simulink model "aircraft_control_model_v2"  (R2020b)
settings: Solver=ode1be  StartTime=0.0  StopTime=t  RelTol=1e-3
values from neighbouring files (symbols this model uses):
  A_ce_CG_14 = A_ce_CG_14(2:3,2:3)    [aircraft_control_model_initialisation_v2.m]
  A_ce_CG_24 = A_ce_CG_24(2:3,2:3)    [aircraft_control_model_initialisation_v2.m]
  A_ce_CG_34 = A_ce_CG_34(2:3,2:3)    [aircraft_control_model_initialisation_v2.m]
  A_sc_CG_10 = A_sc_CG_10(2:3,2:3)    [aircraft_control_model_initialisation_v2.m]
  A_sc_CG_22 = A_sc_CG_22(2:3,2:3)    [aircraft_control_model_initialisation_v2.m]
  A_sc_CG_29 = A_sc_CG_29(2:3,2:3)    [aircraft_control_model_initialisation_v2.m]
  A_sc_CG_36 = A_sc_CG_36(2:3,2:3)    [aircraft_control_model_initialisation_v2.m]
  A_sc_CG_55 = A_sc_CG_55(2:3,2:3)    [aircraft_control_model_initialisation_v2.m]
  actuator_rate = 115*pi/180    (= 2.00712863979)    [aircraft_control_model_initialisation_v2.m]
  ail_sat = 30*pi/180    (= 0.523598775598)    [aircraft_control_model_initialisation_v2.m]
  alpha0 = base_scout_aircraft_constants(16)    [aircraft_control_model_initialisation_v2.m]
  alpha0_ce = base_cessna_aircraft_constants(16)    [aircraft_control_model_initialisation_v2.m]
  alpha0tot_ce_CG_14 = consts_ce_CG_14(17)    [aircraft_control_model_initialisation_v2.m]
  alpha0tot_ce_CG_24 = consts_ce_CG_24(17)    [aircraft_control_model_initialisation_v2.m]
  alpha0tot_ce_CG_34 = consts_ce_CG_34(17)    [aircraft_control_model_initialisation_v2.m]
  alpha0tot_sc_CG_10 = consts_sc_CG_10(17)    [aircraft_control_model_initialisation_v2.m]
  alpha0tot_sc_CG_22 = consts_sc_CG_22(17)    [aircraft_control_model_initialisation_v2.m]
  alpha0tot_sc_CG_29 = consts_sc_CG_29(17)    [aircraft_control_model_initialisation_v2.m]
  alpha0tot_sc_CG_36 = consts_sc_CG_36(17)    [aircraft_control_model_initialisation_v2.m]
  alpha0tot_sc_CG_55 = consts_sc_CG_55(17)    [aircraft_control_model_initialisation_v2.m]
  alpha_ts = base_scout_aircraft_constants(19)    [aircraft_control_model_initialisation_v2.m]
  alpha_ts_ce = base_cessna_aircraft_constants(19)    [aircraft_control_model_initialisation_v2.m]
  alpha_ws = base_scout_aircraft_constants(18)    [aircraft_control_model_initialisation_v2.m]
  alpha_ws_ce = base_cessna_aircraft_constants(18)    [aircraft_control_model_initialisation_v2.m]
  AR_w = base_scout_aircraft_constants(8)    [aircraft_control_model_initialisation_v2.m]
  AR_w_ce = base_cessna_aircraft_constants(8)    [aircraft_control_model_initialisation_v2.m]
  b1 = base_scout_aircraft_constants(23)    [aircraft_control_model_initialisation_v2.m]
  b1_ce = base_cessna_aircraft_constants(23)    [aircraft_control_model_initialisation_v2.m]
  b2 = base_scout_aircraft_constants(24)    [aircraft_control_model_initialisation_v2.m]
  b2_ce = base_cessna_aircraft_constants(24)    [aircraft_control_model_initialisation_v2.m]
  b3 = base_scout_aircraft_constants(25)    [aircraft_control_model_initialisation_v2.m]
  b3_ce = base_cessna_aircraft_constants(25)    [aircraft_control_model_initialisation_v2.m]
  B_ce_CG_14 = B_ce_CG_14(2:3,1:1)    [aircraft_control_model_initialisation_v2.m]
  B_ce_CG_24 = B_ce_CG_24(2:3,1:1)    [aircraft_control_model_initialisation_v2.m]
  B_ce_CG_34 = B_ce_CG_34(2:3,1:1)    [aircraft_control_model_initialisation_v2.m]
  B_sc = B_sc(:,1)    [aircraft_control_model_initialisation_v2.m]
  B_sc_CG_10 = B_sc_CG_10(2:3,1:1)    [aircraft_control_model_initialisation_v2.m]
  B_sc_CG_22 = B_sc_CG_22(2:3,1:1)    [aircraft_control_model_initialisation_v2.m]
  B_sc_CG_29 = B_sc_CG_29(2:3,1:1)    [aircraft_control_model_initialisation_v2.m]
  B_sc_CG_36 = B_sc_CG_36(2:3,1:1)    [aircraft_control_model_initialisation_v2.m]
  B_sc_CG_55 = B_sc_CG_55(2:3,1:1)    [aircraft_control_model_initialisation_v2.m]
  beta_ce_CG_14 = consts_ce_CG_14(21)    [aircraft_control_model_initialisation_v2.m]
  beta_ce_CG_24 = consts_ce_CG_24(21)    [aircraft_control_model_initialisation_v2.m]
  beta_ce_CG_34 = consts_ce_CG_34(21)    [aircraft_control_model_initialisation_v2.m]
  beta_sc_CG_10 = consts_sc_CG_10(21)    [aircraft_control_model_initialisation_v2.m]
  beta_sc_CG_22 = consts_sc_CG_22(21)    [aircraft_control_model_initialisation_v2.m]
  beta_sc_CG_29 = consts_sc_CG_29(21)    [aircraft_control_model_initialisation_v2.m]
  beta_sc_CG_36 = consts_sc_CG_36(21)    [aircraft_control_model_initialisation_v2.m]
  beta_sc_CG_55 = consts_sc_CG_55(21)    [aircraft_control_model_initialisation_v2.m]
  c_e = base_scout_aircraft_constants(10)    [aircraft_control_model_initialisation_v2.m]
  c_e_ce = base_cessna_aircraft_constants(10)    [aircraft_control_model_initialisation_v2.m]
  Cm0 = base_scout_aircraft_constants(11)    [aircraft_control_model_initialisation_v2.m]
  control_surface_feedback = 10    [aircraft_control_model_initialisation_v2.m]
  dCL_w_dalpha = base_scout_aircraft_constants(14)    [aircraft_control_model_initialisation_v2.m]
  dCL_w_dalpha_ce = base_cessna_aircraft_constants(14)    [aircraft_control_model_initialisation_v2.m]
  dCLtot_dalpha = base_scout_aircraft_constants(15)    [aircraft_control_model_initialisation_v2.m]
  dCLtot_dalpha_ce = base_cessna_aircraft_constants(15)    [aircraft_control_model_initialisation_v2.m]
  dt = 1/100    (= 0.01)    [aircraft_control_model_initialisation_v2.m]
  elev_amplitude = 15*pi/180    (= 0.261799387799)    [aircraft_control_model_initialisation_v2.m]
  elev_cutoff = 35*pi/180    (= 0.610865238198)    [aircraft_control_model_initialisation_v2.m]
  elev_period = 1    [aircraft_control_model_initialisation_v2.m]
  elev_period_start = 5    [aircraft_control_model_initialisation_v2.m]
  elev_sat = 28*pi/180    (= 0.488692190558)    [aircraft_control_model_initialisation_v2.m]
  eta_ce_CG_14 = consts_ce_CG_14(22)    [aircraft_control_model_initialisation_v2.m]
  eta_ce_CG_24 = consts_ce_CG_24(22)    [aircraft_control_model_initialisation_v2.m]
  eta_ce_CG_34 = consts_ce_CG_34(22)    [aircraft_control_model_initialisation_v2.m]
  eta_sc_CG_10 = consts_sc_CG_10(22)    [aircraft_control_model_initialisation_v2.m]
  eta_sc_CG_22 = consts_sc_CG_22(22)    [aircraft_control_model_initialisation_v2.m]
  eta_sc_CG_29 = consts_sc_CG_29(22)    [aircraft_control_model_initialisation_v2.m]
  eta_sc_CG_36 = consts_sc_CG_36(22)    [aircraft_control_model_initialisation_v2.m]
  eta_sc_CG_55 = consts_sc_CG_55(22)    [aircraft_control_model_initialisation_v2.m]
  g = base_scout_aircraft_constants(3)    [aircraft_control_model_initialisation_v2.m]
  G = base_scout_aircraft_constants(26)    [aircraft_control_model_initialisation_v2.m]
  g_ce = base_cessna_aircraft_constants(3)    [aircraft_control_model_initialisation_v2.m]
  G_ce = base_cessna_aircraft_constants(26)    [aircraft_control_model_initialisation_v2.m]
  h0 = base_scout_aircraft_constants(13)    [aircraft_control_model_initialisation_v2.m]
  h_cg = base_scout_aircraft_constants(12)    [aircraft_control_model_initialisation_v2.m]
  K = base_scout_aircraft_constants(7)    [aircraft_control_model_initialisation_v2.m]
  l_m = base_scout_aircraft_constants(27)    [aircraft_control_model_initialisation_v2.m]
  l_m_ce = base_cessna_aircraft_constants(27)    [aircraft_control_model_initialisation_v2.m]
  m = base_scout_aircraft_constants(2)    [aircraft_control_model_initialisation_v2.m]
  m_ce = base_cessna_aircraft_constants(2)    [aircraft_control_model_initialisation_v2.m]
  modM = base_scout_aircraft_constants(30)    [aircraft_control_model_initialisation_v2.m]
  modM_ce = base_cessna_aircraft_constants(30)    [aircraft_control_model_initialisation_v2.m]
  n = base_scout_aircraft_constants(1)    [aircraft_control_model_initialisation_v2.m]    (also in xplane_data_decoder.m = data_input(6,2))
  ppgain_actuator_D = 1.076123507883140e+02    (= 107.612350788)    [aircraft_control_model_initialisation_v2.m]
  ppgain_actuator_P = 20.729870007825970    (= 20.7298700078)    [aircraft_control_model_initialisation_v2.m]
  ppgain_D = 0.637114873357555    (= 0.637114873358)    [aircraft_control_model_initialisation_v2.m]
  ppgain_P = -86.717674561182620    (= -86.7176745612)    [aircraft_control_model_initialisation_v2.m]
  r = base_scout_aircraft_constants(29)    [aircraft_control_model_initialisation_v2.m]
  r_ce = base_cessna_aircraft_constants(29)    [aircraft_control_model_initialisation_v2.m]
  rho = base_scout_aircraft_constants(4)    [aircraft_control_model_initialisation_v2.m]
  rho_ce = base_cessna_aircraft_constants(4)    [aircraft_control_model_initialisation_v2.m]
  rud_sat = 28*pi/180    (= 0.488692190558)    [aircraft_control_model_initialisation_v2.m]
  s_e = base_scout_aircraft_constants(9)    [aircraft_control_model_initialisation_v2.m]
  s_e_ce = base_cessna_aircraft_constants(9)    [aircraft_control_model_initialisation_v2.m]
  s_tp = base_scout_aircraft_constants(6)    [aircraft_control_model_initialisation_v2.m]
  s_w = base_scout_aircraft_constants(5)    [aircraft_control_model_initialisation_v2.m]
  s_w_ce = base_cessna_aircraft_constants(5)    [aircraft_control_model_initialisation_v2.m]
  tr = base_scout_aircraft_constants(28)    [aircraft_control_model_initialisation_v2.m]
  tr_ce = base_cessna_aircraft_constants(28)    [aircraft_control_model_initialisation_v2.m]
undefined symbols (not defined in the file or in its folder): A_sc
libraries: simulink x6, pid_lib x4, etargetslib x2, dspnetwork x2, aerolibanimutils x1, sldrtlib x1, cstblocks x1
(part 1 of 3)
settings Model: Creator=declan  LastModifiedBy=declan

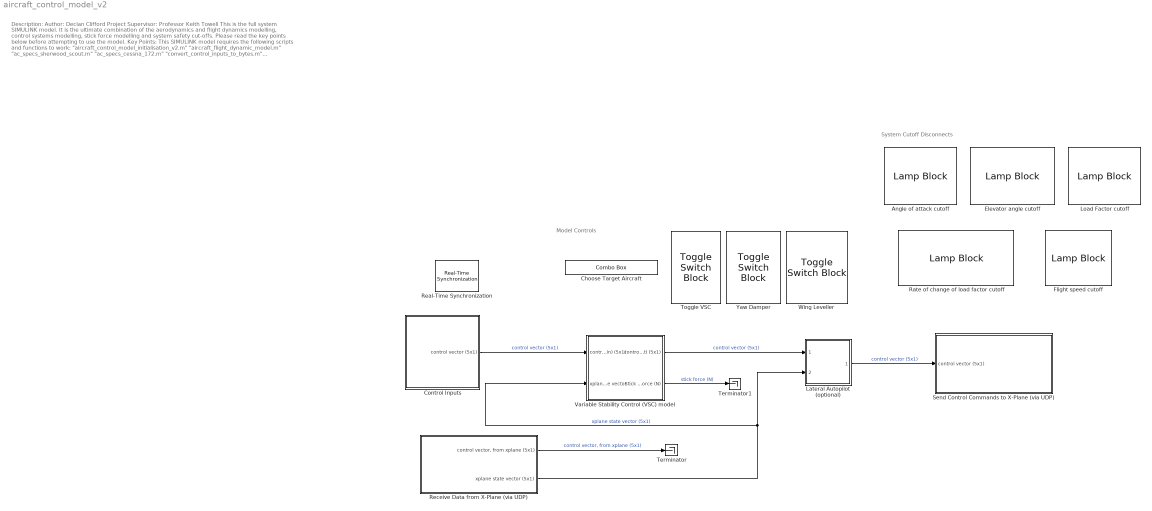
== system aircraft_control_model_v2 ==
  note: Description:
      |
      | Author: Declan Clifford
      | Project Supervisor: Professor Keith Towell
      |
      | This is the full system SIMULINK model. It is the ultimate combination of the aerodynamics and flight dynamics modelling, control systems modelling, stick force modelling and system safety cut-offs.
      |
      | Please read the key points below before attempting to use the model.
      |
      | Key Points:
      |
      | This SIMULINK model requires the following scripts and functions to work:
      | "aircraft_control_model_initialisation_v2.m"
      | "aircraft_flight_dynamic_model.m"
      | "ac_specs_sherwood_scout.m"
      | "ac_specs_cessna_172.m"
      | "convert_control_inputs_to_bytes.m"
      | "elevator_input.m"
      | "flightspeedcutoff.m"
      | "xplane_data_decoder.m"
      |
      | "aircraft_control_model_initialisation_v2" is the SIMULINK model's initialisation script. Please run this script before using the SIMULINK model. It is important the user reads and understand the initialisation script before using the SIMULINK model.
      |
      | "aircraft_flight_dynamic_model" generates the state space matrices required for the flight simulations in this SIMULINK model. It is important the user reads and understands this script before using the SIMULINK model.
      |
      | The model is integrated with X-Plane 11, version 11.52. Connection with X-Plane is performed via UDP. NOTE: USING DIFFERENT VERSIONS OF X-PLANE RUNS THE RISK OF THE RECEIVED DATA REFS BEING INCORRECT, AND SO NONE OF THE RECEIVED DATA FROM X-PLANE WILL BE CORRECT.
      |
      | The X-Plane 11 Sherwood Scout Model can be found at:
      | https://github.com/TheOfficialDarthVader/GDP_52_Variable_Stability_Demonstrator/tree/main/x_plane_sherwood_scout
      | There are three versions of this model; a version with struts, a version without struts and an older "legacy" version of the model.
      |
      | It is recommended to use the wing yaw damper and wing leveller while running X-Plane. This will allow the pilot to forget about lateral aircraft control and focus only on inputting elevator deflections. The throttle will still however need to be controlled to trim the aircraft.
      |
      | The model control inputs are either in the form of a USB joystick or predefined control input. See the "control inputs" block for more details. The joystick inputs for pitch, roll, yaw and the throttle should be quite universal, however the trim tab control has been set up as two button commands. button 6 and button 4.
      |
      | As it stands the model is fully functional, however some parts of it are unfinished. The model is currently tuned to work with only the rear actuator model. A front actuator model has not been integrated with this system. Due to unforeseen delays, the Volz servos front actuator model could not be linearsed and integrated with this system. The full, nonlinearised version of the Volz servos front actuator model slows the system down significantly as it is a separate SIMULINK model and so this was not a viable option.
      |
      | Two of the system safety cut-offs are likewise unfinished. These are the rate of change of load factor cutoff and the flight speed cutoff.
      | The rate of change of load factor cut-off can be implemented as follows:
      | At some time step, determine the rate of change of load factor required to cause the aircraft to exceed the load factor limit in some time interval, chosen as 0.1 seconds here. This is the rate of change of load factor cut-off.
      | In algebraic form this could be expressed as:
      | rate_of_change_of_load_factor_cutoff=(load_factor_limit-present_load_factor)/0.1
      | The rate of change of load factor cut-off currently implemented simply states the rate of change of load factor must not exceed 7.8g/s. The output of this cut-off has been multiplied by a gain of zero, which can be removed when the proper method has been implemeted
      |
      | The flight speed cut-off is half implemented. At present it will only cut-off the control system if the flight speed at a current load factor will cause the aircraft to stall. This is stall under both positive and negative g loading. This should very broadly be expanded to the entire flight envelope. So, if the aircraft's flight speed at the aircraft's current load factor is outside of the flight envelope, or very near it, the system should cut-off. As stated before, this has already been done for the stall limits. It's worth noting that the load factor cut-offs are fully functional and the control system will cut-off at a load factor of 3.8g and -0.5g. This is a separate cut-off to the flight speed cut-off.
  note: Model Controls
  note: System Cutoff Disconnects
  Angle of attack cutoff : LampBlock
  Choose Target Aircraft : ComboBox  LabelPosition=Hide  SelectedLabel=Scout CG 0.2935
      settings: Values={{'Scout CG 0.1', 'Scout CG 0.223', 'Scout CG 0.2935', 'Scout CG 0.364', 'Scout CG 0.55', 'Cessna Forward CG', 'Cessna Centre CG', 'Cessna Aft CG', '>:(', 'F-4C Phantom', 'B-747-100'}, [1 2 3 4 5 6 7 8 9 10 11]}
  Control Inputs : Subsystem  mask{controlvectorselect=Joystick}
      mask prompts: controlvectorselect "Select control method >:("
      mask TypeOptions controlvectorselect: Predefined Input | Joystick
      mask Display: image('control_inputs.JPG'); % Use "Edit Image" on toolstrip to change.
  Elevator angle cutoff : LampBlock
  Flight speed cutoff : LampBlock
  Lateral Autopilot (optional) : Subsystem
      mask Display: image('autopilot_symbol.JPG'); % Use "Edit Image" on toolstrip to change.
  Load Factor cutoff : LampBlock
  Rate of change of load factor cutoff : LampBlock
  Real-Time Synchronization : sldrtlib/Real-Time Synchronization  SampleTime=dt  MaxMissedTicks=500  ShowMissedTicks=off  YieldWhenWaiting=off
  Receive Data from X-Plane (via UDP) : Subsystem
      mask Display: image('udp_receive.JPG'); % Use "Edit Image" on toolstrip to change.
  Send Control Commands to X-Plane (via UDP) : Subsystem
      mask Display: image('udp_send.JPG'); % Use "Edit Image" on toolstrip to change.
  Terminator : Terminator
  Terminator1 : Terminator
  Toggle VSC : ToggleSwitchBlock
      settings: Values={{'Off', 'On'}, [-1 1]}
  Variable Stability Control (VSC) model : Subsystem
      mask Display: image('vsc_cover.JPG'); % Use "Edit Image" on toolstrip to change.
  Wing Leveller : ToggleSwitchBlock
      settings: Values={{'Off', 'On'}, [0 1]}
  Yaw Damper : ToggleSwitchBlock
      settings: Values={{'Off', 'On'}, [0 1]}
  wires:
  Receive Data from X-Plane (via UDP)/2(xplane state vector (5x1)) -> Lateral Autopilot (optional)/2(xplane state vector), Variable Stability Control (VSC) model/2(xplane state vector)  "xplane state vector (5x1)"
  Lateral Autopilot (optional)/1(control vector (output)) -> Send Control Commands to X-Plane (via UDP)/1(control vector (5x1))  "control vector (5x1)"
  Receive Data from X-Plane (via UDP)/1("control vector, from xplane (5x1)") -> Terminator/1  "control vector, from xplane (5x1)"
  Control Inputs/1(control vector (5x1)) -> Variable Stability Control (VSC) model/1(control vector (in) (5x1))  "control vector (5x1)"
  Variable Stability Control (VSC) model/1(control vector (out) (5x1)) -> Lateral Autopilot (optional)/1(control vector (input))  "control vector (5x1)"
  Variable Stability Control (VSC) model/2(Stick Force (N)) -> Terminator1/1  "stick force (N)"

== system aircraft_control_model_v2/Control Inputs ==
  Constant1 : Constant  Value=controlvectorselect
  Switch1 : Switch  Criteria=u2 > Threshold  Threshold=1
  pilot joystick input : Subsystem
  predefined control input : Subsystem
  control vector (5x1) : Outport
  wires:
  pilot joystick input/1(control vector (5x1)) -> Switch1/1  "control vector (5x1)"
  predefined control input/1(control vector (5x1)) -> Switch1/3  "control vector (5x1)"
  Constant1/1 -> Switch1/2
  Switch1/1 -> control vector (5x1)/1  "control vector (5x1)"

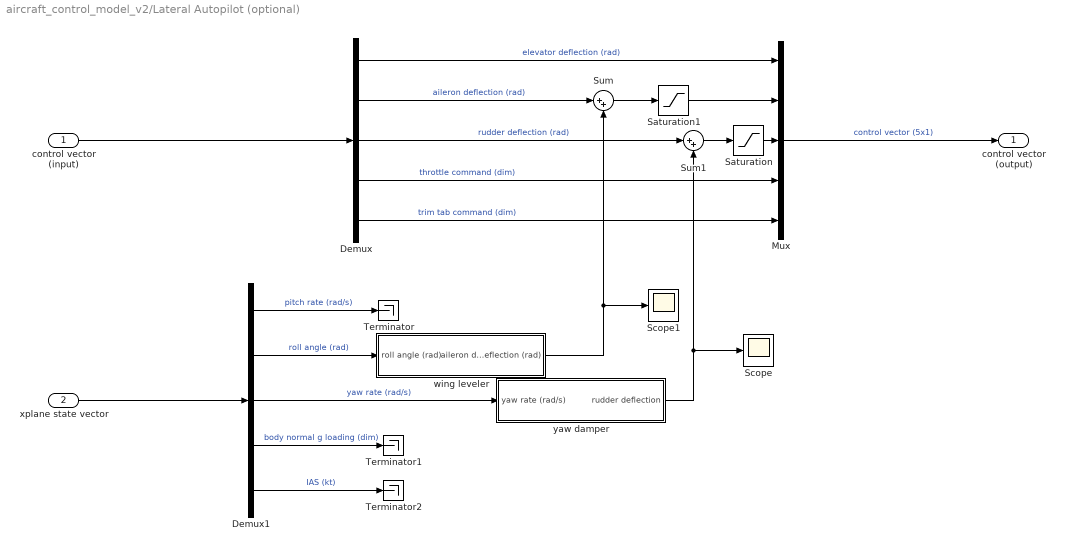
== system aircraft_control_model_v2/Lateral Autopilot (optional) ==
  control vector (input) : Inport
  xplane state vector : Inport  Port=2
  Demux : Demux  Outputs=5
  Demux1 : Demux  Outputs=5
  Mux : Mux  Inputs=5
  Saturation : Saturate  UpperLimit=rud_sat  LowerLimit=-rud_sat
  Saturation1 : Saturate  UpperLimit=ail_sat  LowerLimit=-ail_sat
  Scope : Scope
  Scope1 : Scope
  Sum : Sum  Inputs=|++
  Sum1 : Sum  Inputs=|++
  Terminator : Terminator
  Terminator1 : Terminator
  Terminator2 : Terminator
  wing leveler : Subsystem
  yaw damper : Subsystem
  control vector (output) : Outport
  wires:
  Saturation1/1 -> Mux/2
  Demux1/2 -> wing leveler/1(roll angle (rad))  "roll angle (rad)"
  Demux/4 -> Mux/4  "throttle command (dim)"
  Sum1/1 -> Saturation/1
  Demux1/4 -> Terminator1/1  "body normal g loading (dim)"
  Demux1/1 -> Terminator/1  "pitch rate (rad/s)"
  Sum/1 -> Saturation1/1
  Demux1/3 -> yaw damper/1(yaw rate (rad/s))  "yaw rate (rad/s)"
  Demux/2 -> Sum/1  "aileron deflection (rad)"
  Demux1/5 -> Terminator2/1  "IAS (kt)"
  Saturation/1 -> Mux/3
  Mux/1 -> control vector (output)/1  "control vector (5x1)"
  wing leveler/1(aileron deflection (rad)) -> Scope1/1, Sum/2
  yaw damper/1(rudder deflection) -> Scope/1, Sum1/2
  Demux/1 -> Mux/1  "elevator deflection (rad)"
  Demux/5 -> Mux/5  "trim tab command (dim)"
  Demux/3 -> Sum1/1  "rudder deflection (rad)"
  xplane state vector/1 -> Demux1/1
  control vector (input)/1 -> Demux/1

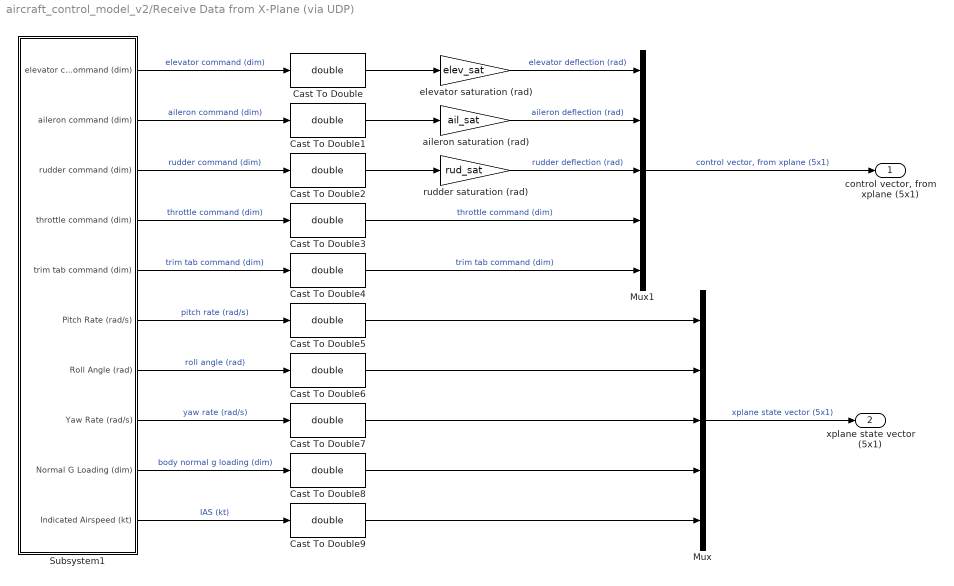
== system aircraft_control_model_v2/Receive Data from X-Plane (via UDP) ==
  Cast To Double{,1..9} (10 alike) : DataTypeConversion  OutDataTypeStr=double
  Mux : Mux  Inputs=5
  Mux1 : Mux  Inputs=5
  Subsystem1 : Subsystem
  aileron saturation (rad) : Gain  Gain=ail_sat
  elevator saturation (rad) : Gain  Gain=elev_sat
  rudder saturation (rad) : Gain  Gain=rud_sat
  "control vector, from xplane (5x1)" : Outport
  xplane state vector (5x1) : Outport  Port=2
  wires:
  Subsystem1/6(Pitch Rate (rad/s)) -> Cast To Double5/1  "pitch rate (rad/s)"
  Subsystem1/2(aileron command (dim)) -> Cast To Double1/1  "aileron command (dim)"
  Cast To Double2/1 -> rudder saturation (rad)/1
  Cast To Double4/1 -> Mux1/5  "trim tab command (dim)"
  Cast To Double3/1 -> Mux1/4  "throttle command (dim)"
  Subsystem1/5(trim tab command (dim)) -> Cast To Double4/1  "trim tab command (dim)"
  rudder saturation (rad)/1 -> Mux1/3  "rudder deflection (rad)"
  Subsystem1/1(elevator command (dim)) -> Cast To Double/1  "elevator command (dim)"
  Cast To Double/1 -> elevator saturation (rad)/1
  Subsystem1/4(throttle command (dim)) -> Cast To Double3/1  "throttle command (dim)"
  Subsystem1/9(Normal G Loading (dim)) -> Cast To Double8/1  "body normal g loading (dim)"
  aileron saturation (rad)/1 -> Mux1/2  "aileron deflection (rad)"
  Subsystem1/3(rudder command (dim)) -> Cast To Double2/1  "rudder command (dim)"
  Subsystem1/8(Yaw Rate (rad/s)) -> Cast To Double7/1  "yaw rate (rad/s)"
  Subsystem1/10(Indicated Airspeed (kt)) -> Cast To Double9/1  "IAS (kt)"
  elevator saturation (rad)/1 -> Mux1/1  "elevator deflection (rad)"
  Subsystem1/7(Roll Angle (rad)) -> Cast To Double6/1  "roll angle (rad)"
  Cast To Double1/1 -> aileron saturation (rad)/1
  Mux/1 -> xplane state vector (5x1)/1  "xplane state vector (5x1)"
  Mux1/1 -> "control vector, from xplane (5x1)"/1  "control vector, from xplane (5x1)"
  Cast To Double9/1 -> Mux/5
  Cast To Double8/1 -> Mux/4
  Cast To Double7/1 -> Mux/3
  Cast To Double6/1 -> Mux/2
  Cast To Double5/1 -> Mux/1

== system aircraft_control_model_v2/Send Control Commands to X-Plane (via UDP) ==
  control vector (5x1) : Inport
  1 byte [0] : Constant  Value=[48]  OutDataTypeStr=uint8
  Demux : Demux  Outputs=5
  MATLAB Function : MATLAB Function  TreatAsAtomicUnit=on
  Pack Bytes : etargetslib/Byte Pack  datatypes={'uint8','uint8','single','single','single'}  byteAlign=1
  Send to X-Plane : dspnetwork/UDP Send  remoteURL='127.0.0.1'  remotePort=49000  localURL='0.0.0.0'  localPortSource=Automatically determine  localPort=-1  sendBufferSize=8192  sampletime=-1  blockPlatform=[]  separateLengthPort=0
  control surface deflections to control surface commands : Subsystem
  wires:
  Demux/3 -> control surface deflections to control surface commands/3(rudder deflection (rad))  "rudder deflection (rad)"
  control vector (5x1)/1 -> Demux/1
  MATLAB Function/4(trim_cmd) -> Pack Bytes/5
  1 byte [0]/1 -> Pack Bytes/2
  Demux/4 -> MATLAB Function/4(throttle)  "throttle command (dim)"
  Demux/5 -> MATLAB Function/5(trimtab)  "trim tab command (dim)"
  MATLAB Function/3(throttle_cmd) -> Pack Bytes/4
  MATLAB Function/1(header) -> Pack Bytes/1
  MATLAB Function/2(control_surfaces_cmd) -> Pack Bytes/3
  Pack Bytes/1 -> Send to X-Plane/1
  control surface deflections to control surface commands/1(elevator) -> MATLAB Function/1(elevator)  "elevator command (dim)"
  Demux/1 -> control surface deflections to control surface commands/1(elevator deflection (rad))  "elevator deflection (rad)"
  Demux/2 -> control surface deflections to control surface commands/2(aileron deflection (rad))  "aileron deflection (rad)"
  control surface deflections to control surface commands/3(rudder) -> MATLAB Function/3(rudder)  "rudder command (dim)"
  control surface deflections to control surface commands/2(aileron) -> MATLAB Function/2(aileron)  "aileron command (dim)"

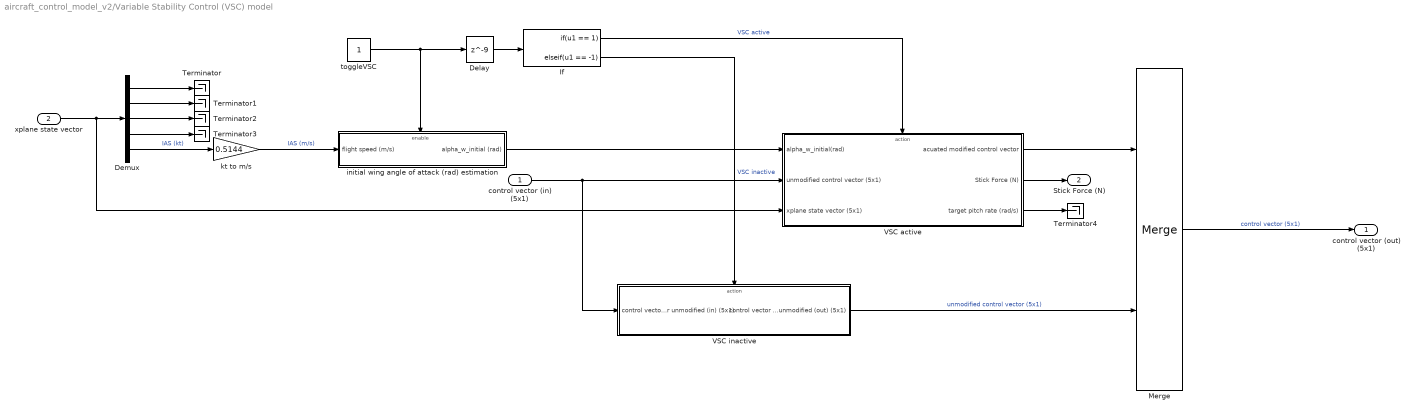
== system aircraft_control_model_v2/Variable Stability Control (VSC) model ==
  control vector (in) (5x1) : Inport
  xplane state vector : Inport  Port=2
  Delay : Delay  DelayLength=9
  Demux : Demux  Outputs=5
  If : If  IfExpression=u1 == 1  ElseIfExpressions=u1 == -1  ShowElse=off
  Merge : Merge
  Terminator{,1..4} (5 alike) : Terminator
  VSC active : Subsystem  TreatAsAtomicUnit=on
  VSC inactive : Subsystem  TreatAsAtomicUnit=on
  initial wing angle of attack (rad) estimation : Subsystem  TreatAsAtomicUnit=on
  kt to m/s : Gain  Gain=0.5144
  toggleVSC : Constant
  control vector (out) (5x1) : Outport
  Stick Force (N) : Outport  Port=2
  wires:
  control vector (in) (5x1)/1 -> VSC inactive/1(control vector unmodified (in) (5x1)), VSC active/2(unmodified control vector (5x1))
  VSC inactive/1(control vector unmodified (out) (5x1)) -> Merge/2  "unmodified control vector (5x1)"
  VSC active/1(acuated modified control vector) -> Merge/1
  Merge/1 -> control vector (out) (5x1)/1  "control vector (5x1)"
  xplane state vector/1 -> VSC active/3(xplane state vector (5x1)), Demux/1
  Demux/1 -> Terminator/1
  Demux/2 -> Terminator1/1
  Demux/3 -> Terminator2/1
  Demux/4 -> Terminator3/1
  Demux/5 -> kt to m/s/1  "IAS (kt)"
  kt to m/s/1 -> initial wing angle of attack (rad) estimation/1(flight speed (m/s))  "IAS (m/s)"
  If/2 -> VSC inactive/Action  "VSC inactive"
  If/1 -> VSC active/Action  "VSC active"
  Delay/1 -> If/1
  toggleVSC/1 -> Delay/1, initial wing angle of attack (rad) estimation/Enable
  initial wing angle of attack (rad) estimation/1(alpha_w_initial (rad)) -> VSC active/1(alpha_w_initial(rad))
  VSC active/2(Stick Force (N)) -> Stick Force (N)/1
  VSC active/3(target pitch rate (rad/s)) -> Terminator4/1

== system aircraft_control_model_v2/Control Inputs/pilot joystick input ==
  If : If  IfExpression=u1 == 32  ElseIfExpressions=u1 == 8
  If Action Subsystem : Subsystem  TreatAsAtomicUnit=on
  If Action Subsystem1 : Subsystem  TreatAsAtomicUnit=on
  If Action Subsystem2 : Subsystem  TreatAsAtomicUnit=on
  Integration with Limits : Integrator  LimitOutput=on  UpperSaturationLimit=1  LowerSaturationLimit=-1
  Merge : Merge  Inputs=3
  Mux : Mux  Inputs=5
  Pilot Joystick All : aerolibanimutils/Pilot Joystick  JoystickID=Joystick1  OutputConfiguration=AllOutputs  SampleTime=dt
  Terminator1 : Terminator
  control surface commands to control surface deflections : Subsystem
  re-ordering control commands : Subsystem
  control vector (5x1) : Outport
  wires:
  re-ordering control commands/1(elevator) -> control surface commands to control surface deflections/1(elevator command (dim))  "elevator command (dim)"
  re-ordering control commands/5(trim tab) -> Mux/5  "trim tab command (dim)"
  control surface commands to control surface deflections/2(aileron deflection (rad)) -> Mux/2  "aileron deflection (rad)"
  re-ordering control commands/3(rudder) -> control surface commands to control surface deflections/3(rudder command (dim))  "rudder command (dim)"
  Pilot Joystick All/3 -> Terminator1/1
  re-ordering control commands/2(aileron) -> control surface commands to control surface deflections/2(aileron command (dim))  "aileron command (dim)"
  control surface commands to control surface deflections/3(rudder deflection (rad)) -> Mux/3  "rudder deflection (rad)"
  control surface commands to control surface deflections/1(elevator deflection (rad)) -> Mux/1  "elevator deflection (rad)"
  re-ordering control commands/4(throttle) -> Mux/4  "throttle command (dim)"
  Pilot Joystick All/1 -> re-ordering control commands/1(analog vector)
  If Action Subsystem1/1(-ve trim tab command) -> Merge/2
  Merge/1 -> Integration with Limits/1
  Pilot Joystick All/2 -> If/1
  If/1 -> If Action Subsystem/Action  "button 6 pressed"
  If Action Subsystem/1(+ve trim tab command) -> Merge/1
  If/3 -> If Action Subsystem2/Action  "no button pressed"
  If Action Subsystem2/1(no trim tab command) -> Merge/3
  If/2 -> If Action Subsystem1/Action  "button 4 pressed"
  Integration with Limits/1 -> re-ordering control commands/2(button vector)  "trim tab command (dim)"
  Mux/1 -> control vector (5x1)/1  "control vector (5x1)"

== system aircraft_control_model_v2/Control Inputs/predefined control input ==
  note: These three blocks create predefined elevator inputs for the model.
      |
      | This is for use when tuning the model and an existing signal's timeseries is required
      |
      | The first block creates an elevator doublet input with period and amplitude controlled in the initialisation script
      |
      | The second block creates a step elevator input
  note: .
  Elevator Doublet Input : Subsystem
  Manual Switch : ManualSwitch
  Mux1 : Mux  Inputs=5
  Step Elevator Input : Constant  Value=elev_amplitude
  aileron : Constant  Value=0
  rudder : Constant  Value=0
  throttle : Constant
  trimtab : Constant  Value=0
  control vector (5x1) : Outport
  wires:
  Step Elevator Input/1 -> Manual Switch/2  "elevator deflection (rad)"
  Manual Switch/1 -> Mux1/1  "elevator deflection (rad)"
  Elevator Doublet Input/1(elevator deflection (rad)) -> Manual Switch/1  "elevator deflection (rad)"
  Mux1/1 -> control vector (5x1)/1  "control vector (5x1)"
  aileron/1 -> Mux1/2  "aileron deflection (rad)"
  throttle/1 -> Mux1/4  "throttle command (dim)"
  rudder/1 -> Mux1/3  "rudder deflection (rad)"
  trimtab/1 -> Mux1/5  "trim tab command (dim)"

== system aircraft_control_model_v2/Lateral Autopilot (optional)/wing leveler ==
  note: Convert data from type double to type single
  note: Convert X-Plane data from type single to type double
  note: Send aileron command to X-Plane via UDP
  roll angle (rad) : Inport
  Cast To Single4 : DataTypeConversion  OutDataTypeStr=single
  Cast to Double : DataTypeConversion  OutDataTypeStr=double
  Constant1 : Constant  Value=0
  PID Controller : pid_lib/PID Controller  Controller=PI  Form=Parallel  TimeDomain=Continuous-time  UseExternalTs=off  SampleTime=-1  IntegratorMethod=Forward Euler  FilterMethod=Forward Euler  ControllerParametersSource=internal  P=0.02  I=0.02  D=0  UseFilter=on  N=100  TunerSelectOption=Transfer Function Based (PID Tuner App)  InitialConditionSource=internal  InitialConditionForIntegrator=0  InitialConditionForFilter=0  DifferentiatorICPrevScaledInput=0  ExternalReset=none  TrackingMode=off  Kt=1  LimitOutput=off  SatLimitsSource=internal  UpperSaturationLimit=inf  LowerSaturationLimit=-inf  LinearizeAsGain=on  AntiWindupMode=none  Kb=1  POutMin=[]  POutMax=[]  IOutMin=[]  IOutMax=[]  DOutMin=[]  DOutMax=[]  NOutMin=[]  NOutMax=[]  SumOutMin=[]  SumOutMax=[]  SaturationOutMin=[]  SaturationOutMax=[]  PParamMin=[]  PParamMax=[]  IParamMin=[]  IParamMax=[]  DParamMin=[]  DParamMax=[]  NParamMin=[]  NParamMax=[]  KbParamMin=[]  KbParamMax=[]  KtParamMin=[]  KtParamMax=[]  KbOutMin=[]  KbOutMax=[]  KtOutMin=[]  KtOutMax=[]  IntegratorOutMin=[]  IntegratorOutMax=[]  FilterOutMin=[]  FilterOutMax=[]  SumI1OutMin=[]  SumI1OutMax=[]  SumI2OutMin=[]  SumI2OutMax=[]  SumI3OutMin=[]  SumI3OutMax=[]  SumI4OutMin=[]  SumI4OutMax=[]  SumDOutMin=[]  SumDOutMax=[]  DifferentiatorOutMin=[]  DifferentiatorOutMax=[]  FilterDiffOutCoefMin=[]  FilterDiffOutCoefMax=[]  ReciprocalOutMin=[]  ReciprocalOutMax=[]  SumDenOutMin=[]  SumDenOutMax=[]  SumNumOutMin=[]  SumNumOutMax=[]  DivideOutMin=[]  DivideOutMax=[]  UdiffTsProdOutMin=[]  UdiffTsProdOutMax=[]  NTsProdOutMin=[]  NTsProdOutMax=[]  UintegralTsProdOutMin=[]  UintegralTsProdOutMax=[]  UngainTsProdOutMin=[]  UngainTsProdOutMax=[]  IntegratorContinuousStateAttributes=''  IntegratorStateMustResolveToSignalObject=off  IntegratorRTWStateStorageClass=Auto  FilterContinuousStateAttributes=''  FilterStateMustResolveToSignalObject=off  FilterRTWStateStorageClass=Auto  ParallelPVariant=InternalParameters  IdealPVariant=Disabled  IVariant=InternalParameters  DVariant=Disabled  IntegratorVariant=Continuous  SatVariant=Disabled  AWVariant=Passthrough  PCopyVariant=Disabled  TRVariant=Disabled  FdbkBlocksVariant=Forward  IdealPFdbkVariant=Disabled  SatFdbkVariant=Disabled  DerivativeFilterVariant=Disabled  NVariant=Disabled  NCopyVariant=Disabled_SignalSpec  FilterICVariant=Disabled  IntegratorICVariant=InternalICs  ExternalResetVariant=Disabled  TRSumVariant=Passthrough  SumFdbkVariant=Disabled  SumVariant=Sum_PI  TsampFilterVariant=InternalTs  TsampNgainVariant=Passthrough  TsampIntegralVariant=Passthrough  ExternalSaturationOutDataTypeStr=Inherit: Same as second input
  Sum1 : Sum  Inputs=|+-
  Switch : Switch  Criteria=u2 > Threshold
  Target Roll Angle (rad) : Constant  Value=0
  toggle_roll_autopilot : Constant
  aileron deflection (rad) : Outport
  wires:
  toggle_roll_autopilot/1 -> Switch/2
  Cast To Single4/1 -> aileron deflection (rad)/1  "aileron deflection (rad)"
  Constant1/1 -> Switch/3
  Sum1/1 -> PID Controller/1
  roll angle (rad)/1 -> Switch/1
  Target Roll Angle (rad)/1 -> Sum1/1
  Switch/1 -> Cast to Double/1
  Cast to Double/1 -> Sum1/2  "Roll Angle (rad)"
  PID Controller/1 -> Cast To Single4/1

== system aircraft_control_model_v2/Lateral Autopilot (optional)/yaw damper ==
  yaw rate (rad/s) : Inport
  Cast To Double1 : DataTypeConversion  OutDataTypeStr=double
  Cast To Single5 : DataTypeConversion  OutDataTypeStr=single
  Constant3 : Constant  Value=0
  PID Controller1 : pid_lib/PID Controller  Controller=PI  Form=Parallel  TimeDomain=Continuous-time  UseExternalTs=off  SampleTime=-1  IntegratorMethod=Forward Euler  FilterMethod=Forward Euler  ControllerParametersSource=internal  P=0.02  I=0.02  D=0  UseFilter=on  N=100  TunerSelectOption=Transfer Function Based (PID Tuner App)  InitialConditionSource=internal  InitialConditionForIntegrator=0  InitialConditionForFilter=0  DifferentiatorICPrevScaledInput=0  ExternalReset=none  TrackingMode=off  Kt=1  LimitOutput=off  SatLimitsSource=internal  UpperSaturationLimit=inf  LowerSaturationLimit=-inf  LinearizeAsGain=on  AntiWindupMode=none  Kb=1  POutMin=[]  POutMax=[]  IOutMin=[]  IOutMax=[]  DOutMin=[]  DOutMax=[]  NOutMin=[]  NOutMax=[]  SumOutMin=[]  SumOutMax=[]  SaturationOutMin=[]  SaturationOutMax=[]  PParamMin=[]  PParamMax=[]  IParamMin=[]  IParamMax=[]  DParamMin=[]  DParamMax=[]  NParamMin=[]  NParamMax=[]  KbParamMin=[]  KbParamMax=[]  KtParamMin=[]  KtParamMax=[]  KbOutMin=[]  KbOutMax=[]  KtOutMin=[]  KtOutMax=[]  IntegratorOutMin=[]  IntegratorOutMax=[]  FilterOutMin=[]  FilterOutMax=[]  SumI1OutMin=[]  SumI1OutMax=[]  SumI2OutMin=[]  SumI2OutMax=[]  SumI3OutMin=[]  SumI3OutMax=[]  SumI4OutMin=[]  SumI4OutMax=[]  SumDOutMin=[]  SumDOutMax=[]  DifferentiatorOutMin=[]  DifferentiatorOutMax=[]  FilterDiffOutCoefMin=[]  FilterDiffOutCoefMax=[]  ReciprocalOutMin=[]  ReciprocalOutMax=[]  SumDenOutMin=[]  SumDenOutMax=[]  SumNumOutMin=[]  SumNumOutMax=[]  DivideOutMin=[]  DivideOutMax=[]  UdiffTsProdOutMin=[]  UdiffTsProdOutMax=[]  NTsProdOutMin=[]  NTsProdOutMax=[]  UintegralTsProdOutMin=[]  UintegralTsProdOutMax=[]  UngainTsProdOutMin=[]  UngainTsProdOutMax=[]  IntegratorContinuousStateAttributes=''  IntegratorStateMustResolveToSignalObject=off  IntegratorRTWStateStorageClass=Auto  FilterContinuousStateAttributes=''  FilterStateMustResolveToSignalObject=off  FilterRTWStateStorageClass=Auto  ParallelPVariant=InternalParameters  IdealPVariant=Disabled  IVariant=InternalParameters  DVariant=Disabled  IntegratorVariant=Continuous  SatVariant=Disabled  AWVariant=Passthrough  PCopyVariant=Disabled  TRVariant=Disabled  FdbkBlocksVariant=Forward  IdealPFdbkVariant=Disabled  SatFdbkVariant=Disabled  DerivativeFilterVariant=Disabled  NVariant=Disabled  NCopyVariant=Disabled_SignalSpec  FilterICVariant=Disabled  IntegratorICVariant=InternalICs  ExternalResetVariant=Disabled  TRSumVariant=Passthrough  SumFdbkVariant=Disabled  SumVariant=Sum_PI  TsampFilterVariant=InternalTs  TsampNgainVariant=Passthrough  TsampIntegralVariant=Passthrough  ExternalSaturationOutDataTypeStr=Inherit: Same as second input
  Sum2 : Sum  Inputs=|+-
  Switch1 : Switch  Criteria=u2 > Threshold
  Target Yaw Rate (rad/s) : Constant  Value=0
  toggle_yaw_autopilot : Constant
  rudder deflection : Outport
  wires:
  Target Yaw Rate (rad/s)/1 -> Sum2/1
  Cast To Single5/1 -> rudder deflection/1  "rudder deflection"
  toggle_yaw_autopilot/1 -> Switch1/2
  yaw rate (rad/s)/1 -> Switch1/1
  Cast To Double1/1 -> Sum2/2  "Yaw Rate (rad/s)"
  Constant3/1 -> Switch1/3
  Switch1/1 -> Cast To Double1/1
  PID Controller1/1 -> Cast To Single5/1
  Sum2/1 -> PID Controller1/1

== system aircraft_control_model_v2/Receive Data from X-Plane (via UDP)/Subsystem1 ==
  Byte Unpack : etargetslib/Byte Unpack  dimensions={5,[9,8]}  datatypes={'uint8','single'}  byteAlign=1
  MATLAB Function : MATLAB Function  TreatAsAtomicUnit=on
  Terminator3 : Terminator
  Terminator4 : Terminator
  UDP Receive : dspnetwork/UDP Receive  localURL='0.0.0.0'  localPort=49004  remoteURL='127.0.0.1'  remotePort=-1  recvBufferSize=8192  dims=293  signalDatatype=uint8  isComplex=off  isVarSize=off  showBlockingTime=off  blockingTime=0  sampletime=dt  blockPlatform=[]
  elevator command (dim) : Outport
  aileron command (dim) : Outport  Port=2
  rudder command (dim) : Outport  Port=3
  throttle command (dim) : Outport  Port=4
  trim tab command (dim) : Outport  Port=5
  Pitch Rate (rad/s) : Outport  Port=6
  Roll Angle (rad) : Outport  Port=7
  Yaw Rate (rad/s) : Outport  Port=8
  Normal G Loading (dim) : Outport  Port=9
  Indicated Airspeed (kt) : Outport  Port=10
  wires:
  UDP Receive/1 -> Byte Unpack/1
  MATLAB Function/10(vInd_kias) -> Indicated Airspeed (kt)/1  "Indicated Airspeed (kt)"
  Byte Unpack/1 -> Terminator4/1  "header"
  MATLAB Function/1(eta) -> elevator command (dim)/1
  Byte Unpack/2 -> MATLAB Function/1(data_input)
  MATLAB Function/9(n) -> Normal G Loading (dim)/1  "Normal G Loading (dim)"
  UDP Receive/2 -> Terminator3/1  "message_length"
  MATLAB Function/6(q) -> Pitch Rate (rad/s)/1  "Pitch Rate (rad/s)"
  MATLAB Function/2(delta_a) -> aileron command (dim)/1
  MATLAB Function/3(delta_r) -> rudder command (dim)/1
  MATLAB Function/7(roll_angle) -> Roll Angle (rad)/1  "Roll Angle (rad)"
  MATLAB Function/8(yaw_rate) -> Yaw Rate (rad/s)/1  "Yaw Rate (rad/s)"
  MATLAB Function/4(throttle) -> throttle command (dim)/1
  MATLAB Function/5(delta_tt) -> trim tab command (dim)/1

== system aircraft_control_model_v2/Send Control Commands to X-Plane (via UDP)/control surface deflections to control surface commands ==
  elevator deflection (rad) : Inport
  aileron deflection (rad) : Inport  Port=2
  rudder deflection (rad) : Inport  Port=3
  Cast To Single : DataTypeConversion  OutDataTypeStr=single
  Cast To Single1 : DataTypeConversion  OutDataTypeStr=single
  Cast To Single2 : DataTypeConversion  OutDataTypeStr=single
  Gain : Gain  Gain=-1/elev_sat
  Gain1 : Gain  Gain=1/ail_sat
  Gain2 : Gain  Gain=1/rud_sat
  elevator : Outport
  aileron : Outport  Port=2
  rudder : Outport  Port=3
  wires:
  Cast To Single2/1 -> elevator/1
  Gain1/1 -> Cast To Single1/1
  Cast To Single/1 -> rudder/1
  Gain/1 -> Cast To Single2/1
  Cast To Single1/1 -> aileron/1
  Gain2/1 -> Cast To Single/1
  elevator deflection (rad)/1 -> Gain/1
  aileron deflection (rad)/1 -> Gain1/1
  rudder deflection (rad)/1 -> Gain2/1

== system aircraft_control_model_v2/Variable Stability Control (VSC) model/VSC active ==
  alpha_w_initial(rad) : Inport
  unmodified control vector (5x1) : Inport  Port=2
  xplane state vector (5x1) : Inport  Port=3
  Action Port : ActionPort  ActionPortLabel=if(u1 == 1)
  Subsystem : Subsystem
  augment elevator input : Subsystem
  rear actuator model : Subsystem
  system safety cutoffs : Subsystem
  target aircraft state space selection : Subsystem
  acuated modified control vector : Outport
  Stick Force (N) : Outport  Port=2
  target pitch rate (rad/s) : Outport  Port=3
  wires:
  unmodified control vector (5x1)/1 -> target aircraft state space selection/2(control vector (5x1)), augment elevator input/5(control vector (5x1))
  augment elevator input/1(modified control vector (5x1)) -> system safety cutoffs/3(modified control vector (5x1)), Subsystem/2(control vector (5x1))
  target aircraft state space selection/3(C_t) -> augment elevator input/3(C_t)
  rear actuator model/1(acuated modified control vector) -> acuated modified control vector/1
  target aircraft state space selection/2(B_t) -> augment elevator input/2(B_t)
  target aircraft state space selection/1(A_t) -> augment elevator input/1(A_t)
  target aircraft state space selection/4(D_t) -> augment elevator input/4(D_t)
  alpha_w_initial(rad)/1 -> system safety cutoffs/2(alpha_w_initial (rad))
  xplane state vector (5x1)/1 -> target aircraft state space selection/1(xplane state vector (5x1)), system safety cutoffs/1(xplane state vector (5x1))
  system safety cutoffs/1(disconnectcontrol?) -> Subsystem/1(disconnectcontrol?)
  Subsystem/1("control vector, out (5x1)") -> rear actuator model/1(modified control vector)
  target aircraft state space selection/5(Stick Force (N)) -> Stick Force (N)/1
  augment elevator input/2(target pitch rate (rad/s)) -> target pitch rate (rad/s)/1

== system aircraft_control_model_v2/Variable Stability Control (VSC) model/VSC inactive ==
  control vector unmodified (in) (5x1) : Inport
  Action Port : ActionPort  ActionPortLabel=elseif(u1 == -1)
  control vector unmodified (out) (5x1) : Outport
  wires:
  control vector unmodified (in) (5x1)/1 -> control vector unmodified (out) (5x1)/1

== system aircraft_control_model_v2/Variable Stability Control (VSC) model/initial wing angle of attack (rad) estimation ==
  flight speed (m/s) : Inport
  Enable : EnablePort
  Constant : Constant  Value=-1
  Constant1 : Constant
  Constant2 : Constant
  Enabled Subsystem : Subsystem  TreatAsAtomicUnit=on
  Gain : Gain  Gain=1/9
  Memory : Memory
  Scope : Scope
  Sum : Sum  Inputs=|++
  Switch : Switch  Criteria=u2 > Threshold  Threshold=9
  alpha_w_initial (rad) : Outport
  wires:
  Switch/1 -> Enabled Subsystem/Enable
  Gain/1 -> Scope/1, alpha_w_initial (rad)/1
  Enabled Subsystem/1(sum of alpha_w_initial (rad)) -> Gain/1
  Constant/1 -> Switch/1
  flight speed (m/s)/1 -> Enabled Subsystem/1(flight speed (m/s))
  Constant2/1 -> Sum/1
  Sum/1 -> Memory/1, Switch/2
  Memory/1 -> Sum/2
  Constant1/1 -> Switch/3

== system aircraft_control_model_v2/Control Inputs/pilot joystick input/If Action Subsystem ==
  Action Port : ActionPort  ActionPortLabel=if(u1 == 32)
  Constant : Constant
  +ve trim tab command : Outport
  wires:
  Constant/1 -> +ve trim tab command/1

== system aircraft_control_model_v2/Control Inputs/pilot joystick input/If Action Subsystem1 ==
  Action Port : ActionPort  ActionPortLabel=elseif(u1 == 8)
  Constant : Constant  Value=-1
  -ve trim tab command : Outport
  wires:
  Constant/1 -> -ve trim tab command/1

== system aircraft_control_model_v2/Control Inputs/pilot joystick input/If Action Subsystem2 ==
  Action Port : ActionPort  ActionPortLabel=else
  Constant : Constant  Value=0
  no trim tab command : Outport
  wires:
  Constant/1 -> no trim tab command/1

== system aircraft_control_model_v2/Control Inputs/pilot joystick input/control surface commands to control surface deflections ==
  elevator command (dim) : Inport
  aileron command (dim) : Inport  Port=2
  rudder command (dim) : Inport  Port=3
  aileron command to aileron deflection : Subsystem
  elevator command to elevator deflection : Subsystem
  rudder command to rudder deflection : Subsystem
  elevator deflection (rad) : Outport
  aileron deflection (rad) : Outport  Port=2
  rudder deflection (rad) : Outport  Port=3
  wires:
  aileron command (dim)/1 -> aileron command to aileron deflection/1(aileron command (dim))
  elevator command to elevator deflection/1(elevator deflection (rad)) -> elevator deflection (rad)/1
  elevator command (dim)/1 -> elevator command to elevator deflection/1(elevator command (dim))
  aileron command to aileron deflection/1(aileron deflection (rad)) -> aileron deflection (rad)/1
  rudder command to rudder deflection/1(rudder deflection (rad)) -> rudder deflection (rad)/1
  rudder command (dim)/1 -> rudder command to rudder deflection/1(rudder command (dim))

== system aircraft_control_model_v2/Control Inputs/pilot joystick input/re-ordering control commands ==
  note: The Pilot Joystick block outputs a signal which varies from -1 to 1 for each of the stick axes and throttle control
  note: Trim tab deflection controlled by button presses for the purposes of this model. Button 6 gives positive trim tab and button 4 gives negative trim tab deflection. The trim tab command is only sent here for convenience to be ordered with the other commands
  analog vector : Inport
  button vector : Inport  Port=2
  Demux1 : Demux  Outputs=6
  Terminator2 : Terminator
  Terminator3 : Terminator
  elevator : Outport
  aileron : Outport  Port=2
  rudder : Outport  Port=3
  throttle : Outport  Port=4
  trim tab : Outport  Port=5
  wires:
  Demux1/6 -> Terminator3/1
  analog vector/1 -> Demux1/1
  Demux1/5 -> Terminator2/1
  Demux1/1 -> aileron/1  "aileron command (dim)"
  Demux1/2 -> elevator/1  "elevator command (dim)"
  Demux1/4 -> rudder/1  "rudder command (dim)"
  Demux1/3 -> throttle/1  "throttle command (dim)"
  button vector/1 -> trim tab/1

== system aircraft_control_model_v2/Control Inputs/predefined control input/Elevator Doublet Input ==
  Clock : Clock
  Constant : Constant  Value=elev_period
  Constant1 : Constant  Value=elev_period_start
  MATLAB Function : MATLAB Function  TreatAsAtomicUnit=on
  Sine Wave : Sin  Amplitude=elev_amplitude  Frequency=2*pi/(elev_period)  SampleTime=0
  elevator deflection (rad) : Outport
  wires:
  Clock/1 -> MATLAB Function/2(clock_time)
  Constant/1 -> MATLAB Function/3(elev_period)
  MATLAB Function/1(u_out) -> elevator deflection (rad)/1  "elevator deflection (rad)"
  Sine Wave/1 -> MATLAB Function/1(u_in)
  Constant1/1 -> MATLAB Function/4(elev_period_start)

== system aircraft_control_model_v2/Variable Stability Control (VSC) model/VSC active/Subsystem ==
  disconnectcontrol? : Inport
  control vector (5x1) : Inport  Port=2
  Demux : Demux  Outputs=5
  Gain : Gain  Gain=control_surface_feedback
  Integrator : Integrator
  Memory : Memory
  Mux : Mux  Inputs=5
  Sum : Sum  Inputs=|+-
  Switch : Switch  Threshold=1
  Switch1 : Switch  Threshold=1
  "control vector, out (5x1)" : Outport
  wires:
  Switch/1 -> Mux/1  "elevator deflection (rad)"
  disconnectcontrol?/1 -> Switch/2, Switch1/2
  Switch1/1 -> Memory/1, Sum/1
  Memory/1 -> Switch1/1
  Gain/1 -> Sum/2
  Integrator/1 -> Gain/1
  Sum/1 -> Switch/1, Integrator/1  "elevator deflection (rad)"
  control vector (5x1)/1 -> Demux/1
  Demux/1 -> Switch1/3, Switch/3  "elevator deflection (rad)"
  Demux/2 -> Mux/2
  Demux/3 -> Mux/3
  Demux/4 -> Mux/4
  Demux/5 -> Mux/5
  Mux/1 -> "control vector, out (5x1)"/1

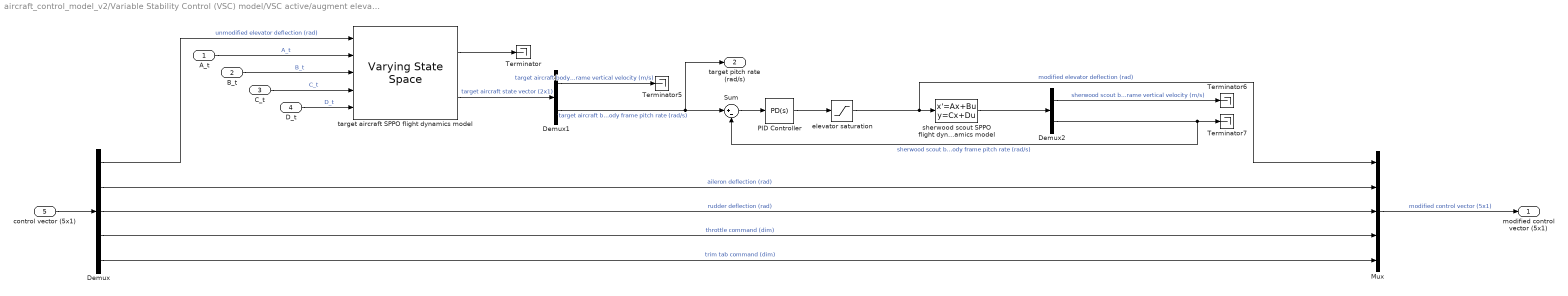
== system aircraft_control_model_v2/Variable Stability Control (VSC) model/VSC active/augment elevator input ==
  A_t : Inport
  B_t : Inport  Port=2
  C_t : Inport  Port=3
  D_t : Inport  Port=4
  control vector (5x1) : Inport  Port=5
  Demux : Demux  Outputs=5
  Demux1 : Demux  Outputs=2
  Demux2 : Demux  Outputs=2
  Mux : Mux  Inputs=5
  PID Controller : pid_lib/PID Controller  Controller=PD  Form=Parallel  TimeDomain=Continuous-time  UseExternalTs=off  SampleTime=-1  IntegratorMethod=Forward Euler  FilterMethod=Forward Euler  ControllerParametersSource=internal  P=ppgain_P  I=0  D=ppgain_D  UseFilter=on  N=100  TunerSelectOption=Transfer Function Based (PID Tuner App)  InitialConditionSource=internal  InitialConditionForIntegrator=0  InitialConditionForFilter=0  DifferentiatorICPrevScaledInput=0  ExternalReset=none  TrackingMode=off  Kt=1  LimitOutput=off  SatLimitsSource=internal  UpperSaturationLimit=inf  LowerSaturationLimit=-inf  LinearizeAsGain=on  AntiWindupMode=none  Kb=1  POutMin=[]  POutMax=[]  IOutMin=[]  IOutMax=[]  DOutMin=[]  DOutMax=[]  NOutMin=[]  NOutMax=[]  SumOutMin=[]  SumOutMax=[]  SaturationOutMin=[]  SaturationOutMax=[]  PParamMin=[]  PParamMax=[]  IParamMin=[]  IParamMax=[]  DParamMin=[]  DParamMax=[]  NParamMin=[]  NParamMax=[]  KbParamMin=[]  KbParamMax=[]  KtParamMin=[]  KtParamMax=[]  KbOutMin=[]  KbOutMax=[]  KtOutMin=[]  KtOutMax=[]  IntegratorOutMin=[]  IntegratorOutMax=[]  FilterOutMin=[]  FilterOutMax=[]  SumI1OutMin=[]  SumI1OutMax=[]  SumI2OutMin=[]  SumI2OutMax=[]  SumI3OutMin=[]  SumI3OutMax=[]  SumI4OutMin=[]  SumI4OutMax=[]  SumDOutMin=[]  SumDOutMax=[]  DifferentiatorOutMin=[]  DifferentiatorOutMax=[]  FilterDiffOutCoefMin=[]  FilterDiffOutCoefMax=[]  ReciprocalOutMin=[]  ReciprocalOutMax=[]  SumDenOutMin=[]  SumDenOutMax=[]  SumNumOutMin=[]  SumNumOutMax=[]  DivideOutMin=[]  DivideOutMax=[]  UdiffTsProdOutMin=[]  UdiffTsProdOutMax=[]  NTsProdOutMin=[]  NTsProdOutMax=[]  UintegralTsProdOutMin=[]  UintegralTsProdOutMax=[]  UngainTsProdOutMin=[]  UngainTsProdOutMax=[]  IntegratorContinuousStateAttributes=''  IntegratorStateMustResolveToSignalObject=off  IntegratorRTWStateStorageClass=Auto  FilterContinuousStateAttributes=''  FilterStateMustResolveToSignalObject=off  FilterRTWStateStorageClass=Auto  ParallelPVariant=InternalParameters  IdealPVariant=Disabled  IVariant=Disabled  DVariant=InternalParameters  IntegratorVariant=Disabled  SatVariant=Disabled  AWVariant=Disabled  PCopyVariant=Disabled  TRVariant=Disabled  FdbkBlocksVariant=Forward  IdealPFdbkVariant=Disabled  SatFdbkVariant=Disabled  DerivativeFilterVariant=ContFilter  NVariant=InternalParameters  NCopyVariant=Disabled  FilterICVariant=InternalICsFilter  IntegratorICVariant=Disabled  ExternalResetVariant=Disabled  TRSumVariant=Passthrough  SumFdbkVariant=Disabled  SumVariant=Sum_PD  TsampFilterVariant=InternalTs  TsampNgainVariant=Passthrough  TsampIntegralVariant=Disabled_SignalSpec  ExternalSaturationOutDataTypeStr=Inherit: Same as second input
  Sum : Sum  Inputs=|+-
  Terminator{,5..7} (4 alike) : Terminator
  elevator saturation : Saturate  UpperLimit=elev_sat  LowerLimit=-elev_sat
  sherwood scout SPPO flight dynamics model : StateSpace  A=A_sc(2:3,2:3)  B=B_sc(2:3)  C=eye(2)  D=zeros(2,1)  InitialCondition=[0;0]
  target aircraft SPPO flight dynamics model : cstblocks/Linear Parameter Varying/Varying State Space  x0=[0;0]  xNames=''  OutputX=on  OutputDX=off
  modified control vector (5x1) : Outport
  target pitch rate (rad/s) : Outport  Port=2
  wires:
  D_t/1 -> target aircraft SPPO flight dynamics model/5  "D_t"
  Demux/1 -> target aircraft SPPO flight dynamics model/1  "unmodified elevator deflection (rad)"
  target aircraft SPPO flight dynamics model/2 -> Demux1/1  "target aircraft state vector (2x1)"
  Demux/4 -> Mux/4  "throttle command (dim)"
  Demux/5 -> Mux/5  "trim tab command (dim)"
  Demux/3 -> Mux/3  "rudder deflection (rad)"
  Demux/2 -> Mux/2  "aileron deflection (rad)"
  C_t/1 -> target aircraft SPPO flight dynamics model/4  "C_t"
  target aircraft SPPO flight dynamics model/1 -> Terminator/1
  A_t/1 -> target aircraft SPPO flight dynamics model/2  "A_t"
  B_t/1 -> target aircraft SPPO flight dynamics model/3  "B_t"
  Demux1/1 -> Terminator5/1  "target aircraft body frame vertical velocity (m/s)"
  control vector (5x1)/1 -> Demux/1
  Demux1/2 -> Sum/1, target pitch rate (rad/s)/1  "target aircraft body frame pitch rate (rad/s)"
  Sum/1 -> PID Controller/1
  PID Controller/1 -> elevator saturation/1
  elevator saturation/1 -> Mux/1, sherwood scout SPPO flight dynamics model/1  "modified elevator deflection (rad)"
  sherwood scout SPPO flight dynamics model/1 -> Demux2/1
  Demux2/1 -> Terminator6/1  "sherwood scout body frame vertical velocity (m/s)"
  Demux2/2 -> Terminator7/1, Sum/2  "sherwood scout body frame pitch rate (rad/s)"
  Mux/1 -> modified control vector (5x1)/1  "modified control vector (5x1)"
